simulink library "nintblocks"  (Simulink 6.0)
settings: Solver=ode45  StartTime=0.0  StopTime=10.0  RelTol=1e-3
libraries: cstblocks x2
settings Model: LastModifiedBy=dvalerio

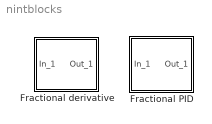
== system nintblocks ==
  Fractional PID : Subsystem  mask(Fractional PID controller){kp=1, kd=1, vd=0.5, ki=1, vi=-0.5, bandwidth=[0.01 100], n=5, form1=crone, exp1=mcltime, decomp1=frac}
      mask prompts: form1 "formula:"; exp1 "expansion:"; decomp1 "decomposition:"
      mask help: Enter expressions for the parameters of function nipid.
      mask init:
      | form2 = {'crone', 'carlson', 'matsuda', 'cfehigh', 'cfelow', 'tustin', 'simpson', '1ofd', '2ofd', '3ofd', 'delta', 'impulse', 'step'};
      | formula = form2{form1};
      | exp2 = {'mcltime', 'mcltimeINV', 'cfe', 'cfeINV'};
      | expansion = exp2{exp1};
      | decomp2 = {'frac', 'all'};
      | decomposition = decomp2{decomp1};
      mask Help: Type 'help nipid' at the command prompt for further help.
      mask StyleString: edit,edit,edit,edit,edit,edit,edit,popup(crone|carlson|matsuda|cfehigh|cfelow|tustin|simpson|1ofd|2ofd|3ofd|delta|impulse|step),popup(mcltime|mcltimeINV|cfe|cfeINV),popup(frac|all)
      mask Display: fprintf('nipid')
  Fractional derivative : Subsystem  mask(Fractional derivative){k=1, v=0.5, bandwidth=[0.01 100], n=5, form1=crone, exp1=mcltime, decomp1=frac}
      mask prompts: form1 "formula:"; exp1 "expansion:"; decomp1 "decomposition:"
      mask help: Enter expressions for the parameters of function nid.
      mask init: same as nintblocks/Fractional PID
      mask Help: Type 'help nid' at the command prompt for further help.
      mask StyleString: edit,edit,edit,edit,popup(crone|carlson|matsuda|cfehigh|cfelow|tustin|simpson|1ofd|2ofd|3ofd|delta|impulse|step),popup(mcltime|mcltimeINV|cfe|cfeINV),popup(frac|all)
      mask Display: fprintf('nid')

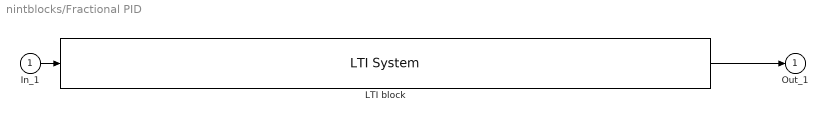
== system nintblocks/Fractional PID ==
  In_1 : Inport  Port=1  LatchInput=off
  LTI block : cstblocks/LTI System  sys=nipid(kp, kd, vd, ki, vi, bandwidth, n, formula, expansion, decomposition)  IC=[]
  Out_1 : Outport  InitialOutput=0
  wires:
  In_1/1 -> LTI block/1
  LTI block/1 -> Out_1/1

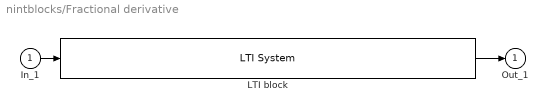
== system nintblocks/Fractional derivative ==
  In_1 : Inport  Port=1  LatchInput=off
  LTI block : cstblocks/LTI System  sys=nid(k, v, bandwidth, n, formula, expansion, decomposition)  IC=[]
  Out_1 : Outport  InitialOutput=0
  wires:
  In_1/1 -> LTI block/1
  LTI block/1 -> Out_1/1
